simulink model "IBVS"  (R2020b)
settings: Solver=VariableStepAuto  StartTime=0.0  StopTime=10  RelTol=1e-3
values from neighbouring files (symbols this model uses):
  dT = 1/frequency    (= 0.005)    [init.m]    (also in init_IBVS.m = 0.002)
  f = 0.5    [init.m]    (also in init_IBVS.m = 0.1)
  init_pose = [C ; ang']    [init.m]    (also in init_IBVS.m = [position(1:3); orientation'])
  Kd = 0*eye(4)    [init.m]    (also in init_IBVS.m)
  Kp = 1*eye(4)    [init.m]    (also in init_IBVS.m = 3*eye(4))
  O = [0; 0; 0]    [init.m]    (also in init_IBVS.m)
  p1 = [1.7; 0.65; 0.1]    [init.m]    (also in init_IBVS.m = [0.5; 0.0; 0.1]; plot_IBVS.m = p_pos(i, 1:3)' + Robj * (p_1 - p_pos(i, 1:3)'))
  p2 = [1.7; 0.85; 0.1]    [init.m]    (also in init_IBVS.m = [0.5; 0.1; 0.1]; plot_IBVS.m = p_pos(i, 1:3)' + Robj * (p_2 - p_pos(i, 1:3)'))
  ref = [ref1; ref2]    [init.m]    (also in init_IBVS.m)
libraries: simulink x1
settings Model: Creator=Acer  LastModifiedBy=antonio

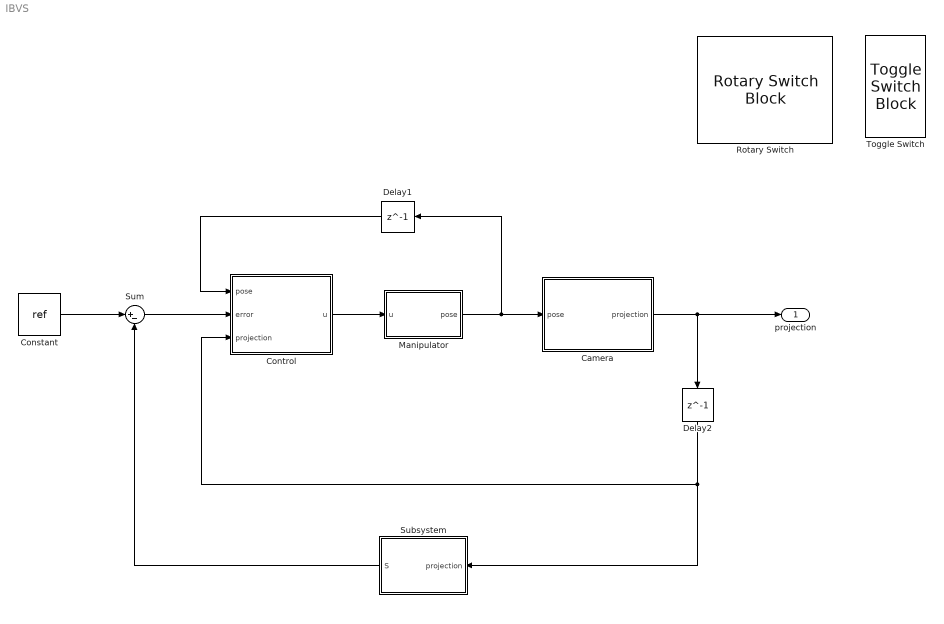
== system IBVS ==
  Camera : Subsystem
  Constant : Constant  Value=ref  SampleTime=-1
  Control : Subsystem
  Delay1 : Delay  DelayLength=1
  Delay2 : Delay  DelayLength=1
  Manipulator : Subsystem
  Rotary Switch : RotarySwitchBlock  LabelPosition=Bottom
      settings: Values={{'Off', 'Low', 'Medium', 'High'}, [0 0.1 0.2 0.3]}
  Subsystem : Subsystem
  Sum : Sum  Inputs=|+-
  Toggle Switch : ToggleSwitchBlock  LabelPosition=Bottom
      settings: Values={{'Off', 'On'}, [0 1]}
  projection : Outport
  wires:
  Camera/1(projection) -> projection/1, Delay2/1
  Delay2/1 -> Control/3(projection), Subsystem/1(projection)
  Delay1/1 -> Control/1(pose)
  Control/1(u) -> Manipulator/1(u)
  Sum/1 -> Control/2(error)
  Manipulator/1(pose) -> Camera/1(pose), Delay1/1
  Constant/1 -> Sum/1
  Subsystem/1(S) -> Sum/2

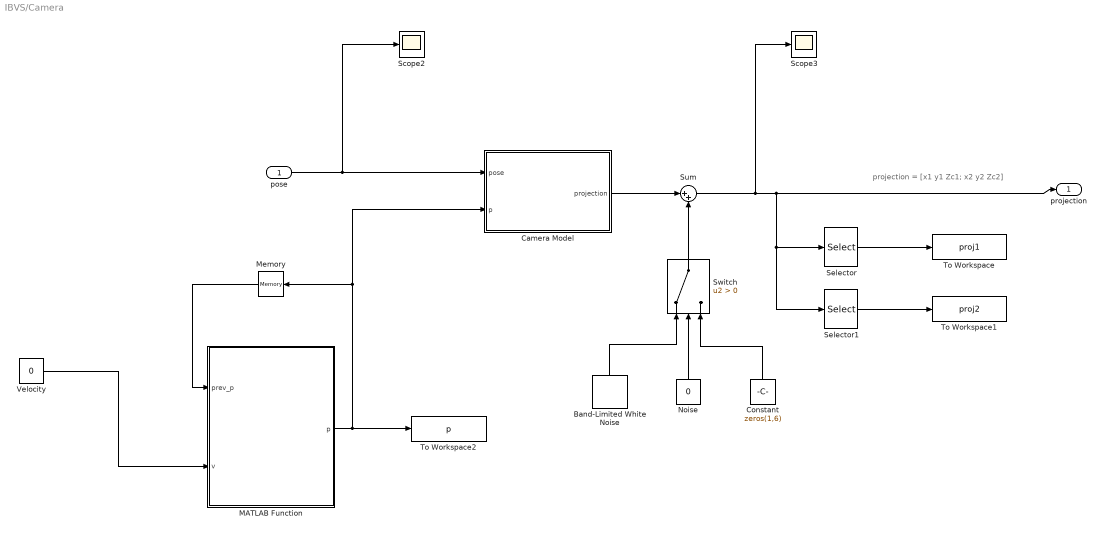
== system IBVS/Camera ==
  note: projection = [x1 y1 Zc1; x2 y2 Zc2]
  pose : Inport
  Band-Limited White Noise : simulink/Sources/Band-Limited White Noise  Cov=[0.00001 0.00001 0.00001 0.00001 0.00001 0.00001]  Ts=0.01  seed=[23341 10 14 19 2123 186]
  Camera Model : MATLAB Function  TreatAsAtomicUnit=on
  Constant : Constant  Value=zeros(1,6)
  MATLAB Function : MATLAB Function  TreatAsAtomicUnit=on  SystemSampleTime=dT
  Memory : Memory  InitialCondition=[p1; p2]
  Noise : Constant  Value=0
  Scope2 : Scope
  Scope3 : Scope
  Selector : Selector  InputPortWidth=6  IndexOptions=Index vector (dialog)  Indices=[1 2]  OutputSizes=1
  Selector1 : Selector  InputPortWidth=6  IndexOptions=Index vector (dialog)  Indices=[4 5]  OutputSizes=1
  Sum : Sum  Inputs=|++
  Switch : Switch  Criteria=u2 > Threshold
  To Workspace : ToWorkspace  VariableName=proj1  SampleTime=0.1
  To Workspace1 : ToWorkspace  VariableName=proj2  SampleTime=0.1
  To Workspace2 : ToWorkspace  VariableName=p  SampleTime=0.1
  Velocity : Constant  Value=0  SampleTime=dT
  projection : Outport
  wires:
  pose/1 -> Scope2/1, Camera Model/1(pose)
  Selector1/1 -> To Workspace1/1
  Selector/1 -> To Workspace/1
  Camera Model/1(projection) -> Sum/1
  Sum/1 -> Scope3/1, projection/1, Selector1/1, Selector/1
  Switch/1 -> Sum/2
  Noise/1 -> Switch/2
  Band-Limited White Noise/1 -> Switch/1
  Constant/1 -> Switch/3
  MATLAB Function/1(p) -> Camera Model/2(p), Memory/1, To Workspace2/1
  Memory/1 -> MATLAB Function/1(prev_p)
  Velocity/1 -> MATLAB Function/2(v)

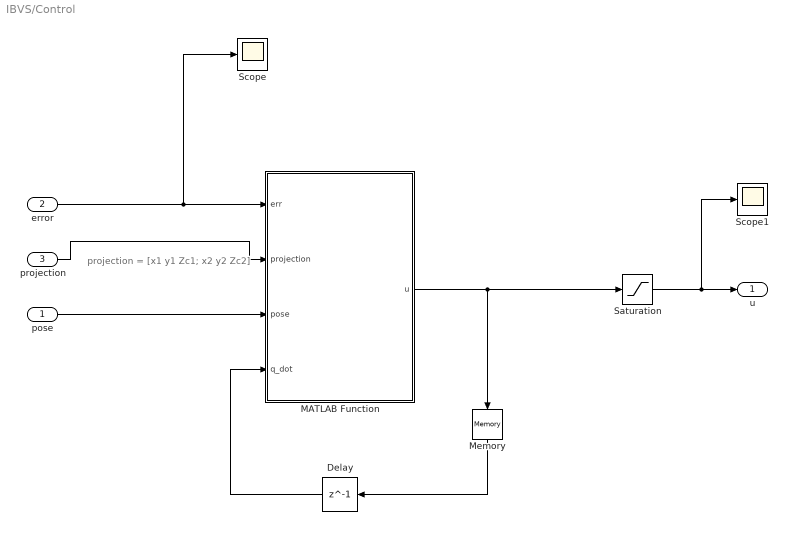
== system IBVS/Control ==
  note: projection = [x1 y1 Zc1; x2 y2 Zc2]
  pose : Inport
  error : Inport  Port=2
  projection : Inport  Port=3
  Delay : Delay  DelayLength=1
  MATLAB Function : MATLAB Function  TreatAsAtomicUnit=on  SystemSampleTime=1/200
  Memory : Memory  InitialCondition=zeros(6,1)
  Saturation : Saturate
  Scope : Scope
  Scope1 : Scope
  u : Outport
  wires:
  error/1 -> Scope/1, MATLAB Function/1(err)
  pose/1 -> MATLAB Function/3(pose)
  Delay/1 -> MATLAB Function/4(q_dot)
  Memory/1 -> Delay/1
  projection/1 -> MATLAB Function/2(projection)
  MATLAB Function/1(u) -> Saturation/1, Memory/1
  Saturation/1 -> Scope1/1, u/1

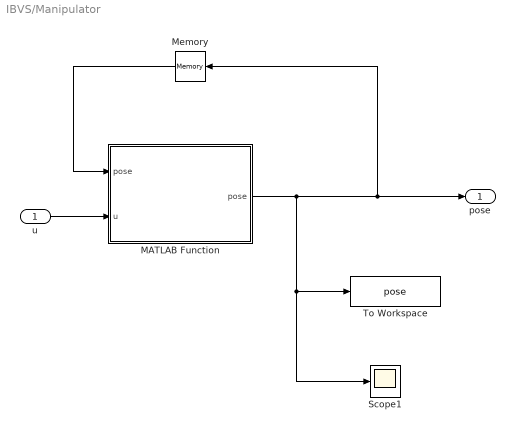
== system IBVS/Manipulator ==
  u : Inport
  MATLAB Function : MATLAB Function  TreatAsAtomicUnit=on  SystemSampleTime=1/200
  Memory : Memory  InitialCondition=init_pose
  Scope1 : Scope
  To Workspace : ToWorkspace  VariableName=pose  SampleTime=0.1
  pose : Outport
  wires:
  u/1 -> MATLAB Function/2(u)
  Memory/1 -> MATLAB Function/1("pose ")
  MATLAB Function/1(pose) -> Scope1/1, To Workspace/1, Memory/1, pose/1

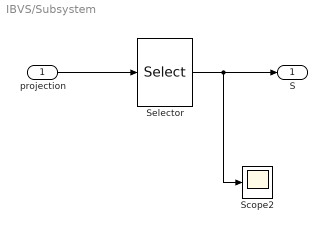
== system IBVS/Subsystem ==
  projection : Inport
  Scope2 : Scope
  Selector : Selector  InputPortWidth=6  IndexOptions=Index vector (dialog)  Indices=[1 2 4 5]  OutputSizes=1
  S : Outport
  wires:
  projection/1 -> Selector/1
  Selector/1 -> Scope2/1, S/1

== matlab function IBVS/Control/MATLAB Function ==
  data: err input; projection input; pose input; Kp parameter; u output; p2 parameter; Kd parameter; q_dot input; p1 parameter
function u = fcn(err, projection, pose, Kp, p2, Kd, q_dot, p1)

% projection = [x1 y1 Zc1; x2 y2 Zc2]
x1 = projection(1);         % x projection in the image plane
y1 = projection(2);         % y projection
Zc1 = projection(3);
x2 = projection(4);
y2 = projection(5);
Zc2 = projection(6);
ang = pose(4:6);  % camera's orientation 

if Zc1 == 0 || isnan(Zc1)
    Zc1 = p1(3)- pose(3);
end

if Zc2 == 0 || isnan(Zc2)
    Zc2 = p2(3) - pose(3);
end

% Interaction matrix 
Ls1 = [ -1/Zc1     0     x1/Zc1     x1*y1    -(1+x1^2)     y1;  
        0       -1/Zc1   y1/Zc1    1+y1^2      -x1*y1     -x1];
    
Ls2 = [ -1/Zc2     0     x2/Zc2     x2*y2    -(1+x2^2)     y2;  
        0       -1/Zc2   y2/Zc2    1+y2^2      -x2*y2     -x2];
    
Ls = [Ls1; Ls2];

% Trasformation
Rx = [1   0       0   ;
      0 cos(ang(1)) -sin(ang(1));
      0 sin(ang(1)) cos(ang(1))];

Ry = [cos(ang(2)) 0 sin(ang(2)) ;
       0     1   0    ;
     -sin(ang(2)) 0 cos(ang(2))];
 
Rz = [cos(ang(3)) -sin(ang(3)) 0;
      sin(ang(3))  cos(ang(3)) 0;
       0      0     1];

Rc = Rz * Ry * Rx;

J2 = [1     sin(ang(1))*tan(ang(2))    cos(ang(1))*tan(ang(2));
      0           cos(ang(1))                  -sin(ang(1));
      0     sin(ang(1))/cos(ang(2))    cos(ang(1))/cos(ang(2)) ];

J = eye(6);  % Jacobian J(q)
  
Jl = Ls * [Rc' zeros(3); zeros(3) J2^-1] * J;

% IBVS control Law
u = pinv(Jl) * (Kp * err - Kd * Jl * q_dot);

== matlab function IBVS/Camera/Camera Model ==
  data: projection output; f parameter; O parameter; pose input; p input
function projection = proj(f, O, pose, p)

d = pose(1:3) - O;    % camera's position in world frame
ang = pose(4:6);      % camera's orientation 
p1 = p(1:3);
p2 = p(4:6);

%%
Rx = [1   0       0   ;
      0 cos(ang(1)) -sin(ang(1));
      0 sin(ang(1)) cos(ang(1))];

Ry = [cos(ang(2)) 0 sin(ang(2)) ;
       0     1   0    ;
     -sin(ang(2)) 0 cos(ang(2))];
 
Rz = [cos(ang(3)) -sin(ang(3)) 0;
      sin(ang(3))  cos(ang(3)) 0;
       0      0     1];


Rc = Rz * Ry * Rx;


Twc = [Rc            d;
      zeros(1,3)     1];

%%
P = diag([f,f,1]) * [eye(3), zeros(3,1)]; % camera projection matrix

p_cam1 = Twc^-1 * [p1; 1];   % point's position in camera frame
p_cam2 = Twc^-1 * [p2; 1];

p_tilde1 = P * p_cam1;
p_tilde2 = P * p_cam2;

x_proj1 = p_tilde1(1)/p_cam1(3);
y_proj1 = p_tilde1(2)/p_cam1(3);
Zc1 = p_cam1(3);

x_proj2 = p_tilde2(1)/p_cam2(3);
y_proj2 = p_tilde2(2)/p_cam2(3);
Zc2 = p_cam2(3);


projection  = [x_proj1; y_proj1; Zc1; x_proj2; y_proj2; Zc2]; %; x_proj2; y_proj2; Zc2];

end

== matlab function IBVS/Manipulator/MATLAB Function ==
  data: pose input; u input; pose output; dT parameter
function pose = fcn(pose, u, dT)

position = zeros(3, 1);
angle = zeros(3, 1);
ang = u(4:6);

Rx = [1   0       0   ;
      0 cos(ang(1)) -sin(ang(1));
      0 sin(ang(1)) cos(ang(1))];

Ry = [cos(ang(2)) 0 sin(ang(2)) ;
       0     1   0    ;
     -sin(ang(2)) 0 cos(ang(2))];
 
Rz = [cos(ang(3)) -sin(ang(3)) 0;
      sin(ang(3))  cos(ang(3)) 0;
       0      0     1];

J1 = Rz * Ry * Rx;

J2 = [1     sin(ang(1))*tan(ang(2))    cos(ang(1))*tan(ang(2));
      0           cos(ang(1))                  -sin(ang(1));
      0     sin(ang(1))/cos(ang(2))    cos(ang(1))/cos(ang(2)) ];


position = pose(1:3) + J1 * u(1:3) * dT;
angle = pose(4:6) + J2 * ang * dT;
pose = [position; angle];

== matlab function IBVS/Camera/MATLAB Function ==
  data: prev_p input; p output; v input; dT parameter
function p = fcn(prev_p ,v, dT)

p1 = prev_p(1:3);
p2 = prev_p(4:6);

p1 = p1 + [0; v; 0] * dT;
p2 = p2 + [0; v; 0] * dT;

p = [p1; p2];
